simulink library "wall_out_IR_radiation"  (R2018b)
settings: Solver=ode45  StartTime=0.0  StopTime=10.0  RelTol=1e-3  EnableMultiTasking=on
undefined symbols (not defined in the file): emission_out
settings Model: Creator=lena.frank  LastModifiedBy=P41573
settings DataIOCC: LimitDataPoints=on  SaveFormat=Array  SignalLoggingSaveFormat=ModelDataLogs
settings OptimizationCC: ExpressionDepthLimit=2147483647  LifeSpan=inf
settings DebuggingCC: UnderspecifiedInitializationDetection=Classic  MergeDetectMultiDrivingBlocksExec=none  SolverPrmCheckMsg=warning  FcnCallInpInsideContextMsg=warning  StateNameClashWarn=warning  SFUnexpectedBacktrackingDiag=warning  SFNoUnconditionalDefaultTransitionDiag=warning  SFExecutionAtInitializationDiag=none
settings HardwareCC: ProdBitPerPointer=32  ProdBitPerSizeT=32  ProdBitPerPtrDiffT=32  ProdLargestAtomicFloat=None  ProdIntDivRoundTo=Undefined  ProdEndianess=Unspecified  ProdWordSize=32  ProdHWDeviceType=32-bit Generic
settings ModelReferenceCC: PropagateSignalLabelsOutOfModel=off
settings SFSimCC: SimUseLocalCustomCode=off
settings RTWCC: RTWUseLocalCustomCode=off
settings CodeAppCC: StateflowObjectComments=on
settings GRTTargetCC: TargetLangStandard=C89/C90 (ANSI)  GeneratePreprocessorConditionals=Disable all  CombineOutputUpdateFcns=off  GRTInterface=on
settings ConfigComp: CovMetricSettings=dw  CovHtmlReporting=on  CovSaveCumulativeToWorkspaceVar=on  CovSaveSingleToWorkspaceVar=on  CovExternalEMLEnable=off

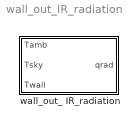
== system wall_out_IR_radiation ==
  wall_out_ IR_radiation : Subsystem

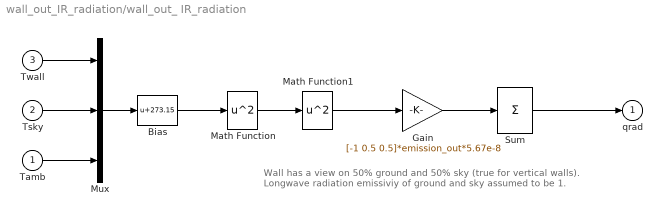
== system wall_out_IR_radiation/wall_out_ IR_radiation ==
  note: Wall has a view on 50% ground and 50% sky (true for vertical walls).
      | Longwave radiation emissiviy of ground and sky assumed to be 1.
  Tamb : Inport
  Tsky : Inport  Port=2
  Twall : Inport  Port=3
  Bias : Bias  Bias=273.15
  Gain : Gain  Gain=[-1 0.5 0.5]*emission_out*5.67e-8
  Math Function : Math  Operator=square  SaturateOnIntegerOverflow=on
  Math Function1 : Math  Operator=square  SaturateOnIntegerOverflow=on
  Mux : Mux  Inputs=3
  Sum : Sum  Inputs=1  SaturateOnIntegerOverflow=on  InputSameDT=on  OutDataTypeStr=Inherit: Same as first input
  qrad : Outport
  wires:
  Math Function1/1 -> Gain/1
  Gain/1 -> Sum/1
  Math Function/1 -> Math Function1/1
  Mux/1 -> Bias/1
  Bias/1 -> Math Function/1
  Twall/1 -> Mux/1
  Sum/1 -> qrad/1
  Tamb/1 -> Mux/3
  Tsky/1 -> Mux/2
